simulink model "untitled"  (R2020b)
settings: Solver=FixedStepAuto  StartTime=0.0  StopTime=10.0  FixedStep=0.02  RelTol=1e-3
settings Model: Creator=GW00216231  LastModifiedBy=GW00216231

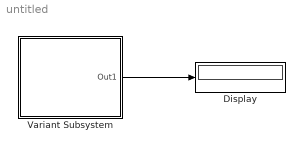
== system untitled ==
  Display : Display
  Variant Subsystem : Subsystem  Variant=on
  wires:
  Variant Subsystem/1(Out1) -> Display/1

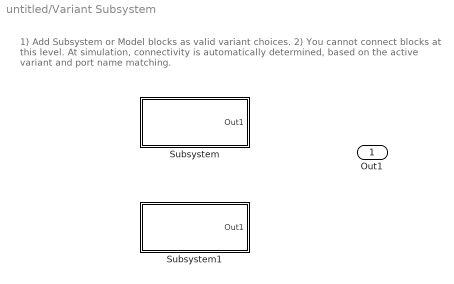
== system untitled/Variant Subsystem ==
  note: 1) Add Subsystem or Model blocks as valid variant choices.
      | 2) You cannot connect blocks at this level. At simulation, connectivity is automatically
      | determined, based on the active variant and port name matching.
  Subsystem : Subsystem  VariantControl=Model ==1
  Subsystem1 : Subsystem  VariantControl=Model ==2
  Out1 : Outport

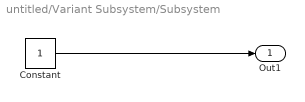
== system untitled/Variant Subsystem/Subsystem ==
  Constant : Constant
  Out1 : Outport
  wires:
  Constant/1 -> Out1/1

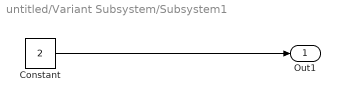
== system untitled/Variant Subsystem/Subsystem1 ==
  Constant : Constant  Value=2
  Out1 : Outport
  wires:
  Constant/1 -> Out1/1
